simulink model "flightController_th"  (R2020a)
settings: Solver=VariableStepAuto  StartTime=0.0  StopTime=10.0  RelTol=1e-3
values from neighbouring files (symbols this model uses):
  BcO = Rx(init_Euler(1))*Ry(init_Euler(2))*Rz(init_Euler(3))    [flightController_ts.m]
  F_aero = [0;0;1000]    [flightController_ts.m]
  init_G_rKite = init_G_rKite + 10*rand(3,1)    [flightController_ts.m]    (also in getInitConditions.m = init_G_rKite.*rotMat)
  init_G_vKite = speed*pathTgt(aBooth,bBooth,meanEl,init_s,1).*rotMat    [getInitConditions.m]
  TcO = Ry(init_El+pi/2)*Rz(init_Az)    [flightController_ts.m]
libraries: flightController_cl x1
settings Model: Creator=Ayaz  LastModifiedBy=Ayaz

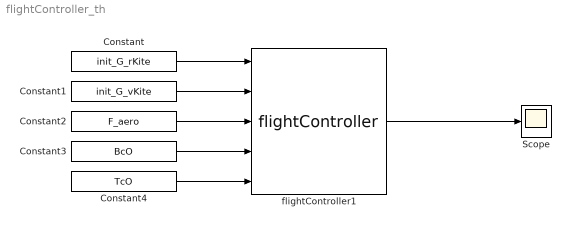
== system flightController_th ==
  Constant : Constant  Value=init_G_rKite
  Constant1 : Constant  Value=init_G_vKite
  Constant2 : Constant  Value=F_aero
  Constant3 : Constant  Value=BcO
  Constant4 : Constant  Value=TcO
  Scope : Scope
  flightController1 : flightController_cl/flightController  PW=pathWidth  PH=pathHeight  PE=pathElev  L1=forwardLen  initialPathParam=initPathVar  kiteMass=mass  kp=aileron_kp  ki=aileron_ki  kd=aileron_kd  tau=aileron_tau
  wires:
  flightController1/1 -> Scope/1
  Constant/1 -> flightController1/1
  Constant1/1 -> flightController1/2
  Constant2/1 -> flightController1/3
  Constant3/1 -> flightController1/4
  Constant4/1 -> flightController1/5
